simulink model "EMA_model_B_PID_tune (1)"  (R2016a)
settings: Solver=VariableStepAuto  StartTime=0.0  StopTime=4  MaxStep=0.01  RelTol=1e-6
undefined symbols (not defined in the file or in its folder): J_a, J_e, J_m, K_C, K_dmp, K_eff, K_emf, K_gs, K_i, K_L, K_md, K_p, K_r, K_t, K_T, N_gear, N_screw, R, R_m, T_L, T_m, V_lim, w_m
libraries: simulink_extras x2, simulink x2
settings Model: Creator=zack.schmid  LastModifiedBy=zack.schmid
settings SolverCC: ZeroCrossAlgorithm=Adaptive
settings DataIOCC: LimitDataPoints=on  SaveOutput=off  SaveTime=off
settings OptimizationCC: ExpressionDepthLimit=2147483647  LifeSpan=1
settings DebuggingCC: UnderspecifiedInitializationDetection=Classic  MergeDetectMultiDrivingBlocksExec=none  MaxConsecutiveZCsMsg=warning  FcnCallInpInsideContextMsg=EnableAllAsWarning  AllowSymbolicDim=off  StateNameClashWarn=warning
settings GRTTargetCC: CombineOutputUpdateFcns=off  GRTInterface=on

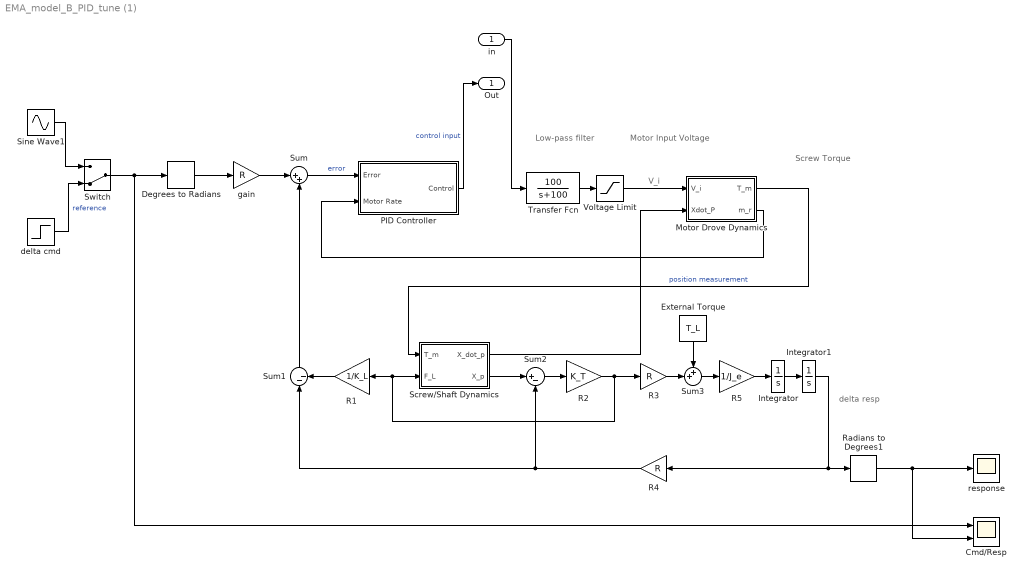
== system EMA_model_B_PID_tune (1) ==
  note: Low-pass
      | filter
  note: Screw
      | Torque
  note: Motor Input
      | Voltage
  note: delta resp
  note: V_i
  in : Inport
  " Switch" : ManualSwitch  CurrentSetting=0
  Cmd/Resp : Scope  NumInputPorts=2
  Degrees to Radians : simulink_extras/Transformations/Degrees to Radians
  External Torque : Constant  Value=T_L
  Integrator : Integrator
  Integrator1 : Integrator
  Motor Drove Dynamics : Subsystem
  PID Controller : Subsystem
  R1 : Gain  Gain=1/K_L
  R2 : Gain  Gain=K_T
  R3 : Gain  Gain=R
  R4 : Gain  Gain=R
  R5 : Gain  Gain=1/J_e
  Radians to Degrees1 : simulink_extras/Transformations/Radians to Degrees
  Screw/Shaft Dynamics : Subsystem
  Sine Wave1 : Sin  Amplitude=0.5  Frequency=8*2*pi  SampleTime=0
  Sum : Sum  Inputs=|++
  Sum1 : Sum  Inputs=|--
  Sum2 : Sum  Inputs=|+-
  Sum3 : Sum  Inputs=++|
  Transfer Fcn : TransferFcn  Numerator=[100]  Denominator=[1 100]
  Voltage Limit : Saturate  UpperLimit=V_lim  LowerLimit=-V_lim  ZeroCross=off
  delta cmd : Step  Time=0  After=10  SampleTime=0  ZeroCross=off
  gain : Gain  Gain=R
  response : Scope
  Out : Outport
  wires:
  Sum/1 -> PID Controller/1(Error)  "error"
  gain/1 -> Sum/1
  Transfer Fcn/1 -> Voltage Limit/1
  Voltage Limit/1 -> Motor Drove Dynamics/1(V_i)
  Sum1/1 -> Sum/2
  R1/1 -> Sum1/2
  Screw/Shaft Dynamics/2(X_p) -> Sum2/1
  Sum2/1 -> R2/1
  R2/1 -> R1/1, Screw/Shaft Dynamics/2(F_L), R3/1
  R3/1 -> Sum3/2
  External Torque/1 -> Sum3/1
  Sum3/1 -> R5/1
  Motor Drove Dynamics/1(T_m) -> Screw/Shaft Dynamics/1(T_m)  "position measurement"
  Screw/Shaft Dynamics/1(X_dot_p) -> Motor Drove Dynamics/2(Xdot_P)
  Integrator/1 -> Integrator1/1
  R5/1 -> Integrator/1
  R4/1 -> Sum2/2, Sum1/1
  Motor Drove Dynamics/2(m_r) -> PID Controller/2(Motor Rate)
  Integrator1/1 -> R4/1, Radians to Degrees1/1
  Radians to Degrees1/1 -> Cmd/Resp/2, response/1
  Degrees to Radians/1 -> gain/1
  Sine Wave1/1 -> " Switch"/1
  " Switch"/1 -> Cmd/Resp/1, Degrees to Radians/1
  delta cmd/1 -> " Switch"/2  "reference"
  PID Controller/1(Control) -> Out/1  "control input"
  in/1 -> Transfer Fcn/1

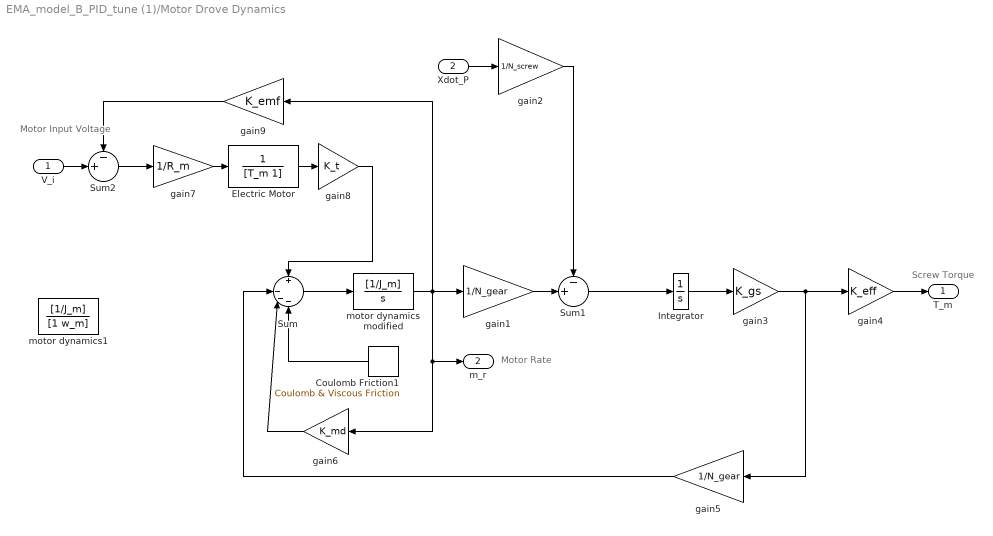
== system EMA_model_B_PID_tune (1)/Motor Drove Dynamics ==
  note: Motor Input
      | Voltage
  note: Motor Rate
  note: Screw Torque
  V_i : Inport
  Xdot_P : Inport  Port=2
  Coulomb Friction1 : simulink/Discontinuities/Coulomb & Viscous Friction  offset=[K_C]  gain=0
  Electric Motor : TransferFcn  Denominator=[T_m 1]
  Integrator : Integrator
  Sum : Sum  Inputs=+|---
  Sum1 : Sum  Inputs=-+|
  Sum2 : Sum  Inputs=-+|
  gain1 : Gain  Gain=1/N_gear
  gain2 : Gain  Gain=1/N_screw
  gain3 : Gain  Gain=K_gs
  gain4 : Gain  Gain=K_eff
  gain5 : Gain  Gain=1/N_gear
  gain6 : Gain  Gain=K_md
  gain7 : Gain  Gain=1/R_m
  gain8 : Gain  Gain=K_t
  gain9 : Gain  Gain=K_emf
  motor dynamics modified : TransferFcn  Numerator=[1/J_m]  Denominator=[1 0]
  motor dynamics1 : TransferFcn  Numerator=[1/J_m]  Denominator=[1 w_m]
  T_m : Outport
  m_r : Outport  Port=2
  wires:
  Sum/1 -> motor dynamics modified/1
  motor dynamics modified/1 -> gain6/1, m_r/1, gain9/1, gain1/1
  Xdot_P/1 -> gain2/1
  gain1/1 -> Sum1/2
  gain2/1 -> Sum1/1
  Sum1/1 -> Integrator/1
  Integrator/1 -> gain3/1
  gain3/1 -> gain5/1, gain4/1
  gain4/1 -> T_m/1
  gain5/1 -> Sum/2
  gain6/1 -> Sum/3
  Coulomb Friction1/1 -> Sum/4
  gain7/1 -> Electric Motor/1
  Electric Motor/1 -> gain8/1
  gain8/1 -> Sum/1
  Sum2/1 -> gain7/1
  gain9/1 -> Sum2/1
  V_i/1 -> Sum2/2

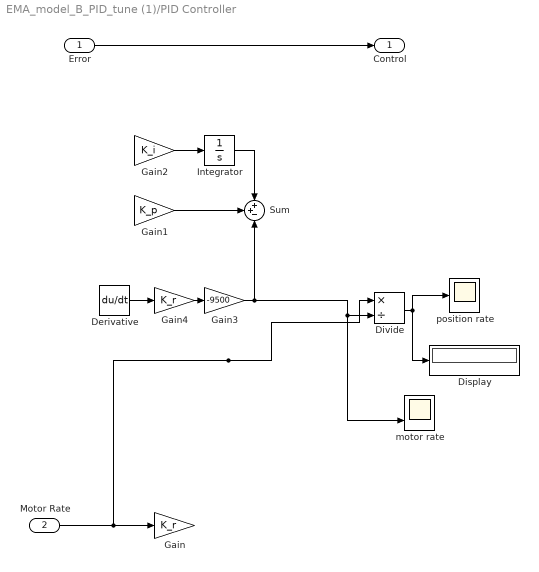
== system EMA_model_B_PID_tune (1)/PID Controller ==
  Error : Inport
  Motor Rate : Inport  Port=2
  Derivative : Derivative
  Display : Display
  Divide : Product  Inputs=*/
  Gain : Gain  Gain=K_r
  Gain1 : Gain  Gain=K_p
  Gain2 : Gain  Gain=K_i
  Gain3 : Gain  Gain=-9500
  Gain4 : Gain  Gain=K_r
  Integrator : Integrator
  Sum : Sum  Inputs=++-
  motor rate : Scope  NumInputPorts=2
  position rate : Scope
  Control : Outport
  wires:
  Motor Rate/1 -> Divide/1, Gain/1
  Gain2/1 -> Integrator/1
  Gain1/1 -> Sum/2
  Integrator/1 -> Sum/1
  Divide/1 -> Display/1, position rate/1
  Gain3/1 -> Sum/3, Divide/2, motor rate/2
  Gain4/1 -> Gain3/1
  Derivative/1 -> Gain4/1
  Error/1 -> Control/1

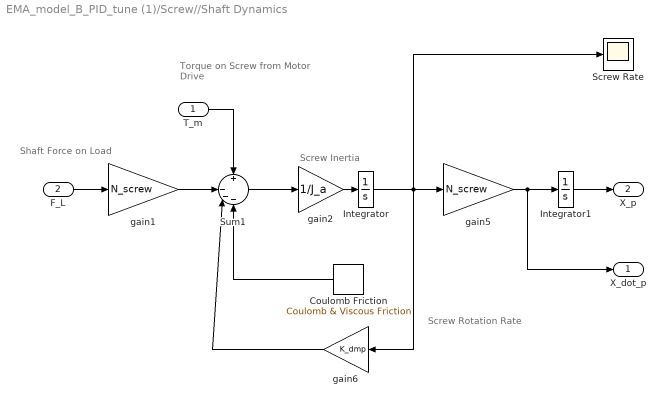
== system EMA_model_B_PID_tune (1)/Screw//Shaft Dynamics ==
  note: Screw Inertia
  note: Screw
      | Rotation
      | Rate
  note: Shaft Force
      | on Load
  note: Torque on Screw
      | from Motor Drive
  T_m : Inport
  F_L : Inport  Port=2
  Coulomb Friction : simulink/Discontinuities/Coulomb & Viscous Friction  offset=[K_C]  gain=0
  Integrator : Integrator  ZeroCross=off
  Integrator1 : Integrator
  Screw Rate : Scope
  Sum1 : Sum  Inputs=+|---
  gain1 : Gain  Gain=N_screw
  gain2 : Gain  Gain=1/J_a
  gain5 : Gain  Gain=N_screw
  gain6 : Gain  Gain=K_dmp
  X_dot_p : Outport
  X_p : Outport  Port=2
  wires:
  Sum1/1 -> gain2/1
  T_m/1 -> Sum1/1
  gain5/1 -> Integrator1/1, X_dot_p/1
  gain2/1 -> Integrator/1
  gain1/1 -> Sum1/2
  F_L/1 -> gain1/1
  gain6/1 -> Sum1/3
  Integrator1/1 -> X_p/1
  Coulomb Friction/1 -> Sum1/4
  Integrator/1 -> Screw Rate/1, gain6/1, gain5/1
